simulink model "full_total_adder"  (R2018b)
settings: Solver=VariableStepAuto  StartTime=0.0  StopTime=10.0  RelTol=1e-3
settings Model: Creator=annat  LastModifiedBy=annat

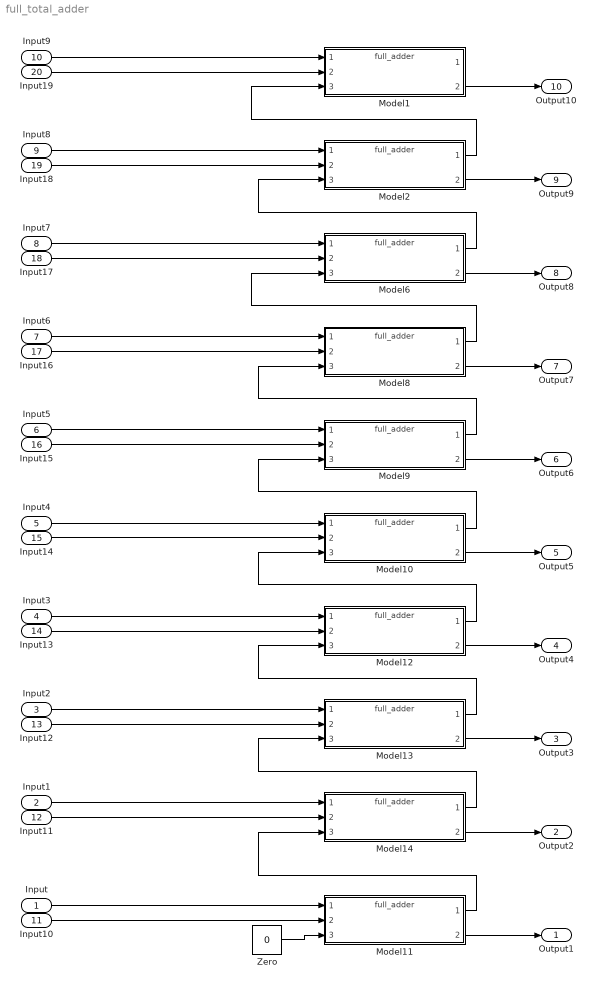
== system full_total_adder ==
  Input : Inport
  Input1 : Inport  Port=2
  Input2 : Inport  Port=3
  Input3 : Inport  Port=4
  Input4 : Inport  Port=5
  Input5 : Inport  Port=6
  Input6 : Inport  Port=7
  Input7 : Inport  Port=8
  Input8 : Inport  Port=9
  Input9 : Inport  Port=10
  Input10 : Inport  Port=11
  Input11 : Inport  Port=12
  Input12 : Inport  Port=13
  Input13 : Inport  Port=14
  Input14 : Inport  Port=15
  Input15 : Inport  Port=16
  Input16 : Inport  Port=17
  Input17 : Inport  Port=18
  Input18 : Inport  Port=19
  Input19 : Inport  Port=20
  Model{1..2,6,8..14} (10 alike) : ModelReference  ModelNameDialog=full_adder  SimulationMode=Normal  ModelReferenceVersion=1.1
  Zero : Constant  Value=0  OutDataTypeStr=Inherit: Inherit via back propagation
  Output1 : Outport
  Output2 : Outport  Port=2
  Output3 : Outport  Port=3
  Output4 : Outport  Port=4
  Output5 : Outport  Port=5
  Output6 : Outport  Port=6
  Output7 : Outport  Port=7
  Output8 : Outport  Port=8
  Output9 : Outport  Port=9
  Output10 : Outport  Port=10
  wires:
  Model8/1 -> Model6/3
  Model9/1 -> Model8/3
  Model10/1 -> Model9/3
  Model12/1 -> Model10/3
  Model13/1 -> Model12/3
  Model14/1 -> Model13/3
  Model6/2 -> Output8/1
  Model8/2 -> Output7/1
  Model9/2 -> Output6/1
  Model10/2 -> Output5/1
  Model12/2 -> Output4/1
  Model13/2 -> Output3/1
  Model14/2 -> Output2/1
  Model11/1 -> Model14/3
  Model11/2 -> Output1/1
  Model2/2 -> Output9/1
  Model6/1 -> Model2/3
  Model1/2 -> Output10/1
  Model2/1 -> Model1/3
  Input10/1 -> Model11/2
  Input11/1 -> Model14/2
  Input/1 -> Model11/1
  Input1/1 -> Model14/1
  Input12/1 -> Model13/2
  Input2/1 -> Model13/1
  Input13/1 -> Model12/2
  Input3/1 -> Model12/1
  Input14/1 -> Model10/2
  Input4/1 -> Model10/1
  Input5/1 -> Model9/1
  Input15/1 -> Model9/2
  Input16/1 -> Model8/2
  Input6/1 -> Model8/1
  Input17/1 -> Model6/2
  Input7/1 -> Model6/1
  Input18/1 -> Model2/2
  Input8/1 -> Model2/1
  Input19/1 -> Model1/2
  Input9/1 -> Model1/1
  Zero/1 -> Model11/3
